simulink model "HexaMotor_Pendulum2"  (R2022b)
settings: Solver=FixedStepAuto  StartTime=0.0  StopTime=inf  RelTol=1e-3  EnableMultiTasking=on
model workspace (MAT data in the model file):
  sampleRate = 0.01
libraries: eeGeneralControl x4, simulink_extras x3, arduinomotorcarrierlib x3, simulink x1
settings Model: ExtModeTrigDuration=2  Creator=bkhusain  LastModifiedBy=arkad
settings SolverCC: AlgebraicLoopSolver=TrustRegion
settings DataIOCC: ReturnWorkspaceOutputs=off
settings OptimizationCC: EnhancedBackFolding=on  PassReuseOutputArgsThreshold=0  MaxStackSize=64  OptimizeBlockOrder=speed  DifferentSizesBufferReuse=on  OptimizationCustomize=off
settings DebuggingCC: ParameterOverflowMsg=none  ParameterUnderflowMsg=error  ParameterPrecisionLossMsg=none  ParameterTunabilityLossMsg=error  UnconnectedInputMsg=warning  UnconnectedOutputMsg=warning  UnconnectedLineMsg=warning  SFMachineParentedDataDiag=warning
settings HardwareCC: ProdBitPerPointer=32  ProdBitPerSizeT=32  ProdBitPerPtrDiffT=32  ProdLargestAtomicInteger=Long  ProdLargestAtomicFloat=Double  ProdWordSize=32  ProdHWDeviceType=ARM Compatible->ARM Cortex
settings ModelReferenceCC: EnableRefExpFcnMdlSchedulingChecks=on
settings SFSimCC: MATLABDynamicMemAlloc=off
settings RTWCC: Description=Embedded Coder  SystemTargetFile=ert.tlc  HardwareBoard=Arduino MKRZero  TLCOptions=-aInlineSetEventsForThisBaseRateFcn=TLC_FALSE -aSuppressMultiTaskScheduler=TLC_FALSE -aRateBasedStepFcn=1  TemplateMakefile=ert_default_tmf  Toolchain=Arduino ARM  BuildConfiguration=Faster Runs  DLArmComputeVersion=19.05
settings CodeAppCC: ForceParamTrailComments=on  OperatorAnnotations=on
settings ERTTargetCC: ERTCustomFileBanners=off  SupportContinuousTime=on  SupportNonInlinedSFcns=on  RemoveResetFunc=off  SupportVariableSizeSignals=on  ModelStepFunctionPrototypeControlCompliant=off  ExtModeTransport=3  ExtModeStaticAlloc=on  ExtModeAutomaticAllocSize=off  ExtModeStaticAllocSize=8192  ExtModeMexFile=ext_xcp  ExtModeIntrfLevel=Level2 - Open

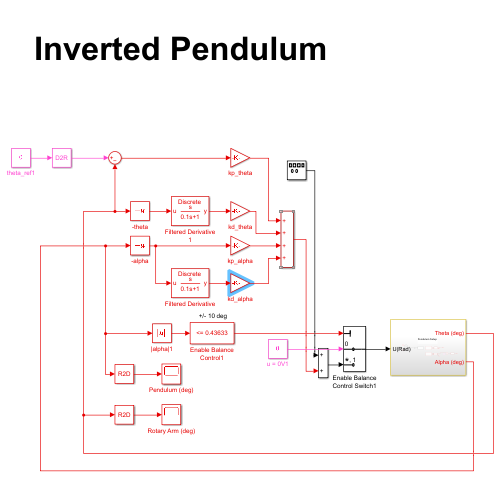
[thumbnail: Simulink's stored preview of the top-level diagram]
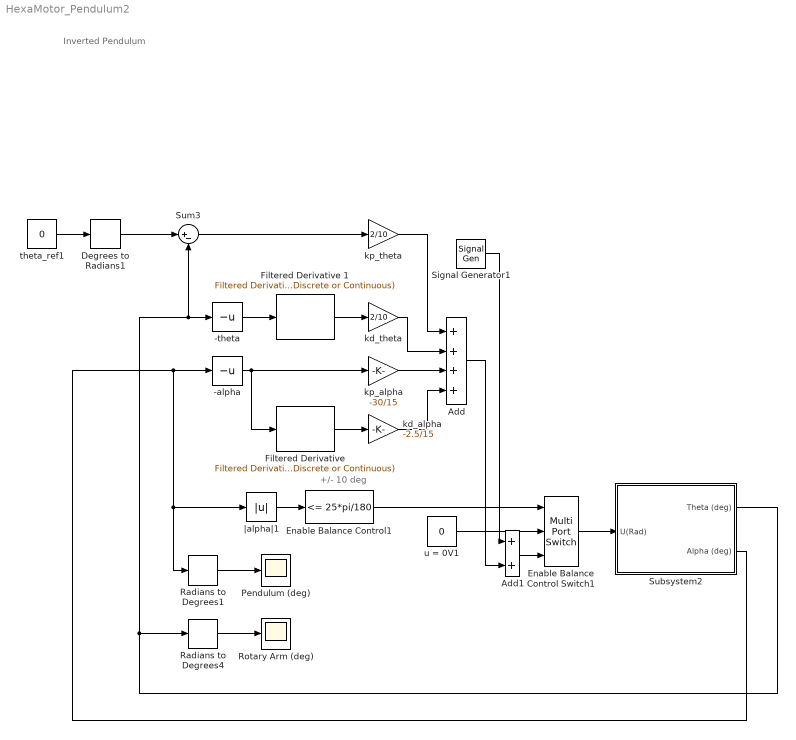
== system HexaMotor_Pendulum2 ==
  note: Inverted Pendulum
  note: +/- 10 deg
  -alpha : UnaryMinus
  -theta : UnaryMinus
  Add : Sum  Inputs=++++
  Add1 : Sum
  Degrees to Radians1 : simulink_extras/Transformations/Degrees to Radians
  Enable Balance Control Switch1 : MultiPortSwitch  DataPortOrder=Zero-based contiguous  Inputs=2  zeroidx=on  SaturateOnIntegerOverflow=off  InputSameDT=off
  Enable Balance Control1 : simulink/Logic and Bit Operations/Compare To Constant  relop=<=  const=25*pi/180  OutDataTypeStr=uint8  ZeroCross=off
  "Filtered Derivative " : eeGeneralControl/Filtered Derivative (Discrete or Continuous)  K=1  T=0.1  B=inf  A=-inf  minRatio=10  init_option=Inherited from block input  x0=0  Ts=-1
  Filtered Derivative 1 : eeGeneralControl/Filtered Derivative (Discrete or Continuous)  K=1  T=0.1  B=inf  A=-inf  minRatio=10  init_option=Inherited from block input  x0=0  Ts=-1
  Pendulum (deg) : Scope
  Radians to Degrees1 : simulink_extras/Transformations/Radians to Degrees
  Radians to Degrees4 : simulink_extras/Transformations/Radians to Degrees
  Rotary Arm (deg) : Scope
  Signal Generator1 : SignalGenerator  Amplitude=0.15  Frequency=15
  Subsystem2 : Subsystem
  Sum3 : Sum  Inputs=|+-
  kd_alpha : Gain  Gain=-2.5/15
  kd_theta : Gain  Gain=2/10
  kp_alpha : Gain  Gain=-30/15
  kp_theta : Gain  Gain=2/10
  theta_ref1 : Constant  Value=0
  u = 0V1 : Constant  Value=0
  |alpha|1 : Abs  SaturateOnIntegerOverflow=off
  wires:
  |alpha|1/1 -> Enable Balance Control1/1
  Degrees to Radians1/1 -> Sum3/1
  Subsystem2/1(Theta (deg)) -> -theta/1, Sum3/2, Radians to Degrees4/1
  Radians to Degrees4/1 -> Rotary Arm (deg)/1
  kd_alpha/1 -> Add/4
  Sum3/1 -> kp_theta/1
  kd_theta/1 -> Add/2
  "Filtered Derivative "/1 -> kd_alpha/1
  Enable Balance Control1/1 -> Enable Balance Control Switch1/1
  -alpha/1 -> "Filtered Derivative "/1, kp_alpha/1
  -theta/1 -> Filtered Derivative 1/1
  kp_theta/1 -> Add/1
  Subsystem2/2(Alpha (deg)) -> Radians to Degrees1/1, |alpha|1/1, -alpha/1
  Radians to Degrees1/1 -> Pendulum (deg)/1
  kp_alpha/1 -> Add/3
  Filtered Derivative 1/1 -> kd_theta/1
  u = 0V1/1 -> Enable Balance Control Switch1/2
  Enable Balance Control Switch1/1 -> Subsystem2/1(U(Rad))
  theta_ref1/1 -> Degrees to Radians1/1
  Signal Generator1/1 -> Add1/1
  Add1/1 -> Enable Balance Control Switch1/3
  Add/1 -> Add1/2

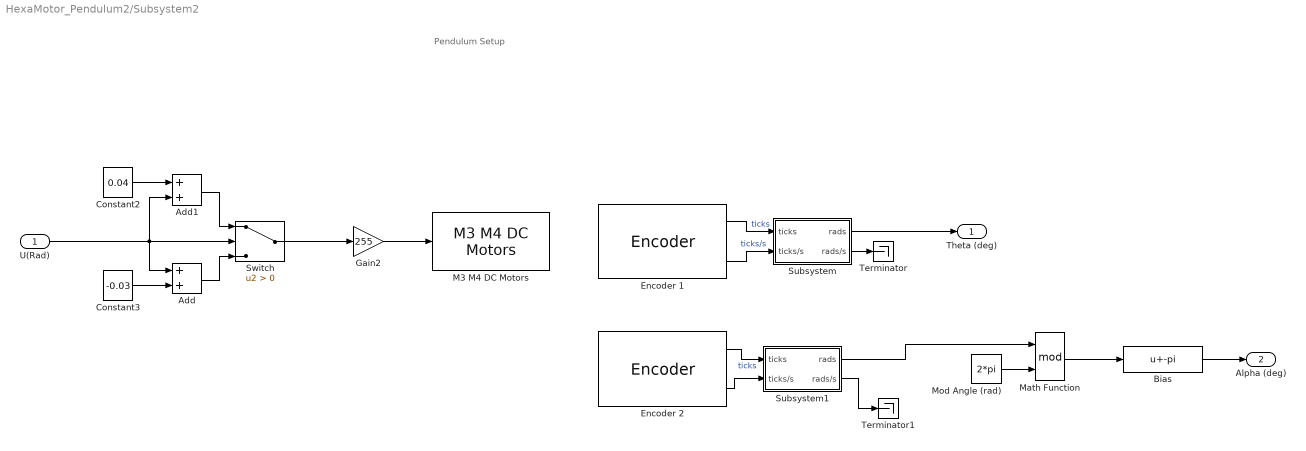
== system HexaMotor_Pendulum2/Subsystem2 ==
  note: Pendulum Setup
  U(Rad) : Inport
  Add : Sum
  Add1 : Sum
  Bias : Bias  Bias=-pi  SaturateOnIntegerOverflow=off
  Constant2 : Constant  Value=0.04  SampleTime=sampleRate
  Constant3 : Constant  Value=-0.03  SampleTime=sampleRate
  Encoder 1 : arduinomotorcarrierlib/Encoder  SlaveAddress=uint8( hex2dec( '66' ) )  blockPlatform=ARDUINO  Encoder=1  ShowSpeed=on  ResetOption=on  SampleTime=sampleRate
  Encoder 2 : arduinomotorcarrierlib/Encoder  SlaveAddress=uint8( hex2dec( '66' ) )  blockPlatform=ARDUINO  Encoder=2  ShowSpeed=on  ResetOption=on  SampleTime=sampleRate
  Gain2 : Gain  Gain=255
  M3 M4 DC Motors : arduinomotorcarrierlib/M3 M4 DC Motors  MotorNumber=M3  forwardPinNumber=3  reversePinNumber=2
  Math Function : Math  Operator=mod  SignedPower=on
  Mod Angle (rad) : Constant  Value=2*pi
  Subsystem : Subsystem
  Subsystem1 : Subsystem
  Switch : Switch  Criteria=u2 > Threshold  SaturateOnIntegerOverflow=off  InputSameDT=off
  Terminator : Terminator
  Terminator1 : Terminator
  Theta (deg) : Outport
  Alpha (deg) : Outport  Port=2
  wires:
  Subsystem/2(rads/s) -> Terminator/1
  Switch/1 -> Gain2/1
  Encoder 1/2 -> Subsystem/2(ticks/s)  "ticks/s"
  Encoder 1/1 -> Subsystem/1(ticks)  "ticks"
  Gain2/1 -> M3 M4 DC Motors/1
  Subsystem/1(rads) -> Theta (deg)/1
  Subsystem1/2(rads/s) -> Terminator1/1
  Encoder 2/1 -> Subsystem1/1(ticks)  "ticks"
  Encoder 2/2 -> Subsystem1/2(ticks/s)
  Bias/1 -> Alpha (deg)/1
  Mod Angle (rad)/1 -> Math Function/2
  Math Function/1 -> Bias/1
  Subsystem1/1(rads) -> Math Function/1
  Add1/1 -> Switch/1
  Constant3/1 -> Add/2
  Add/1 -> Switch/3
  U(Rad)/1 -> Add/1, Add1/2, Switch/2
  Constant2/1 -> Add1/1

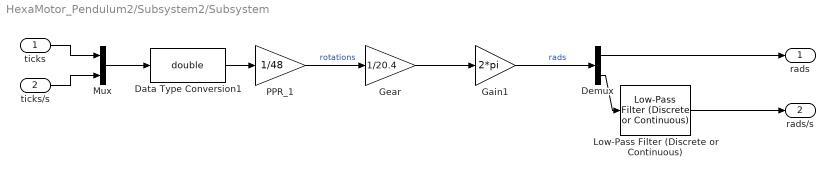
== system HexaMotor_Pendulum2/Subsystem2/Subsystem ==
  ticks : Inport
  ticks/s : Inport  Port=2
  Data Type Conversion1 : DataTypeConversion  OutDataTypeStr=double  SaturateOnIntegerOverflow=off  RndMeth=Floor
  Demux : Demux  Outputs=2
  Gain1 : Gain  Gain=2*pi
  Gear : Gain  Gain=1/20.4
  Low-Pass Filter (Discrete or Continuous) : eeGeneralControl/Low-Pass Filter (Discrete or Continuous)  K=1  T=0.1  B=inf  A=-inf  init_option=Inherited from block input  x0=0  Ts=sampleRate
  Mux : Mux  Inputs=2
  PPR_1 : Gain  Gain=1/48
  rads : Outport
  rads/s : Outport  Port=2
  wires:
  PPR_1/1 -> Gear/1  "rotations"
  Data Type Conversion1/1 -> PPR_1/1
  Mux/1 -> Data Type Conversion1/1
  ticks/1 -> Mux/1
  Gear/1 -> Gain1/1
  ticks/s/1 -> Mux/2
  Gain1/1 -> Demux/1  "rads"
  Demux/1 -> rads/1
  Demux/2 -> Low-Pass Filter (Discrete or Continuous)/1
  Low-Pass Filter (Discrete or Continuous)/1 -> rads/s/1

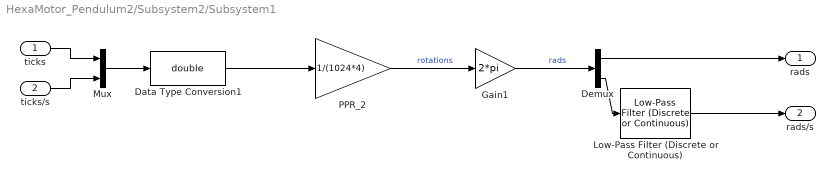
== system HexaMotor_Pendulum2/Subsystem2/Subsystem1 ==
  ticks : Inport
  ticks/s : Inport  Port=2
  Data Type Conversion1 : DataTypeConversion  OutDataTypeStr=double  SaturateOnIntegerOverflow=off  RndMeth=Floor
  Demux : Demux  Outputs=2
  Gain1 : Gain  Gain=2*pi
  Low-Pass Filter (Discrete or Continuous) : eeGeneralControl/Low-Pass Filter (Discrete or Continuous)  K=1  T=0.1  B=inf  A=-inf  init_option=Inherited from block input  x0=0  Ts=sampleRate
  Mux : Mux  Inputs=2
  PPR_2 : Gain  Gain=1/(1024*4)
  rads : Outport
  rads/s : Outport  Port=2
  wires:
  Data Type Conversion1/1 -> PPR_2/1
  Mux/1 -> Data Type Conversion1/1
  ticks/1 -> Mux/1
  ticks/s/1 -> Mux/2
  Gain1/1 -> Demux/1  "rads"
  Demux/1 -> rads/1
  Demux/2 -> Low-Pass Filter (Discrete or Continuous)/1
  Low-Pass Filter (Discrete or Continuous)/1 -> rads/s/1
  PPR_2/1 -> Gain1/1  "rotations"
